simulink model "Lab5"  (R2020b)
settings: Solver=VariableStepAuto  StartTime=0.0  StopTime=10.0  RelTol=1e-3
settings Model: Creator=MY lenovo  LastModifiedBy=MY lenovo

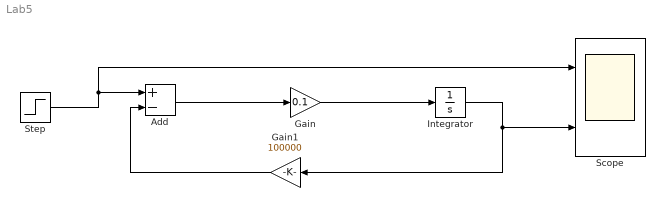
== system Lab5 ==
  Add : Sum  Inputs=+-
  Gain : Gain  Gain=0.1
  Gain1 : Gain  Gain=100000
  Integrator : Integrator
  Scope : Scope  NumInputPorts=2
  Step : Step  SampleTime=0
  wires:
  Add/1 -> Gain/1
  Gain/1 -> Integrator/1
  Step/1 -> Scope/1, Add/1
  Gain1/1 -> Add/2
  Integrator/1 -> Gain1/1, Scope/2
